simulink model "P702_NI_SoftECU"  (R2019a)
settings: Solver=ode1  StartTime=0.0  StopTime=Inf  FixedStep=0.001  RelTol=1e-3  EnableMultiTasking=on
PreLoadFcn:
  | run '.\VeriStand_BlockSet\NIVeriStandAddPaths.m'
undefined symbols (not defined in the file or in its folder): magnitude
libraries: simulink x83, simulink_extras x1
(part 1 of 76)
settings Model: Creator=HILTEST  LastModifiedBy=MSHI15
settings DataIOCC: LimitDataPoints=on  SaveFormat=Array  ReturnWorkspaceOutputs=off
settings OptimizationCC: BlockReduction=off  OptimizeBlockIOStorage=off  BufferReuse=off  GlobalBufferReuse=off  ExpressionFolding=off  LocalBlockOutputs=off  LifeSpan=inf  OptimizeDataStoreBuffers=off  BusAssignmentInplaceUpdate=off
settings DebuggingCC: InheritedTsInSrcMsg=none  RootOutportRequireBusObject=error  PregeneratedLibrarySubsystemCodeDiagnostic=none  StrictBusMsg=ErrorOnBusTreatedAsVector  SFUnexpectedBacktrackingDiag=warning  SFNoUnconditionalDefaultTransitionDiag=warning  SFExecutionAtInitializationDiag=none  ArithmeticOperatorsInVariantConditions=warning
settings HardwareCC: ProdBitPerPointer=32  ProdBitPerSizeT=32  ProdBitPerPtrDiffT=32  ProdLargestAtomicFloat=None  ProdWordSize=32  ProdHWDeviceType=Intel->x86/Pentium  TargetIntDivRoundTo=Zero  TargetEndianess=LittleEndian  TargetHWDeviceType=Generic->Custom
settings ModelReferenceCC: PropagateSignalLabelsOutOfModel=off
settings SFSimCC: SimUseLocalCustomCode=off
settings RTWCC: SystemTargetFile=NIVeriStand.tlc  TemplateMakefile=NIVeriStand_vc.tmf  Description=NI Phar Lap Real-Time & Windows Targets  RTWUseLocalCustomCode=off
settings CodeAppCC: StateflowObjectComments=on
settings STFCustomTargetCC: GeneratePreprocessorConditionals=Disable all  MatFileLogging=on  MATLABClassNameForMDSCustomization=Simulink.SoftwareTarget.TargetSpecificTriggerConfigurationBase  SystemTargetFile=NIVeriStand.tlc
settings ConfigComp: CovMetricSettings=dw  CovHtmlReporting=on  CovSaveCumulativeToWorkspaceVar=on  CovSaveSingleToWorkspaceVar=on  CovExternalEMLEnable=off

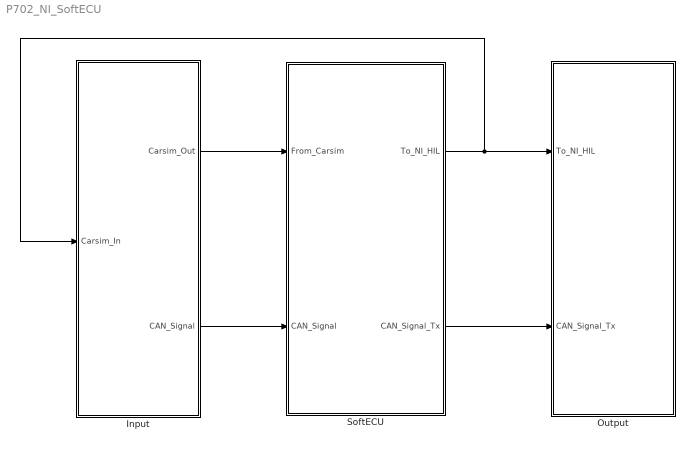
== system P702_NI_SoftECU ==
  Input : Subsystem
  Output : Subsystem
  SoftECU : Subsystem
  wires:
  SoftECU/1(To_NI_HIL) -> Input/1(Carsim_In), Output/1(To_NI_HIL)
  Input/1(Carsim_Out) -> SoftECU/1(From_Carsim)
  Input/2(CAN_Signal) -> SoftECU/2(CAN_Signal)
  SoftECU/2(CAN_Signal_Tx) -> Output/2(CAN_Signal_Tx)

== system P702_NI_SoftECU/Input ==
  Carsim_In : Inport
  ABS_ESC : Subsystem
  ABS_ESC_Disable : S-Function  Priority=1  FunctionName=NIVeriStandIO  Parameters=width dtype portnum stime stype btype  SFunctionDeploymentMode=off  EnableBusSupport=off  mask(NI VeriStand Inport){portnum=1, width=-1, stime=-1, dtype=auto, stype=auto, btype=1}
      mask prompts: portnum "Port number:"; width "Port dimensions (-1 for dynamically sized):"; stime "Sample time (-1 for inherited):"; dtype "Data type:"; stype "Signal type:"; btype "Block type:"
      mask help: Use this inport on any level of nested subsystems to allow NI VeriStand software to map signals to it.
      mask init:
      | NIVeriStandIO_init;
      settings: CopyFcn=NIVeriStand_MDL_functions('', 'IO_copy');  DeleteFcn=NIVeriStand_MDL_functions('', 'IO_delete');  MoveFcn=set_param(gcb, 'Mask', 'on');
      mask Callback portnum: NIVeriStand_MDL_functions('', 'IO_setportnum');
      mask TypeOptions dtype: auto | double | single | int8 | uint8 | int16 | uint16 | int32 | uint32 | boolean
      mask Callback dtype: NIVeriStand_MDL_functions('', 'IO_booleansignal');
      mask TypeOptions stype: auto | real | complex
      mask Display:
      | patch([-x x], [-y y], [.90980 .81960 .32156]);
      | plot([xrad -x x xrad], [yrad -y y yrad]);
      | fprintf('NI In%d', portnum);
  ADAS_Disable : S-Function  Priority=4  FunctionName=NIVeriStandIO  Parameters=width dtype portnum stime stype btype  SFunctionDeploymentMode=off  EnableBusSupport=off  mask(NI VeriStand Inport){portnum=4, width=-1, stime=-1, dtype=auto, stype=auto, btype=1}
      mask prompts: portnum "Port number:"; width "Port dimensions (-1 for dynamically sized):"; stime "Sample time (-1 for inherited):"; dtype "Data type:"; stype "Signal type:"; btype "Block type:"
      mask help: Use this inport on any level of nested subsystems to allow NI VeriStand software to map signals to it.
      mask init:
      | NIVeriStandIO_init;
      settings: CopyFcn=NIVeriStand_MDL_functions('', 'IO_copy');  DeleteFcn=NIVeriStand_MDL_functions('', 'IO_delete');  MoveFcn=set_param(gcb, 'Mask', 'on');
      mask Callback portnum: NIVeriStand_MDL_functions('', 'IO_setportnum');
      mask TypeOptions dtype: auto | double | single | int8 | uint8 | int16 | uint16 | int32 | uint32 | boolean
      mask Callback dtype: NIVeriStand_MDL_functions('', 'IO_booleansignal');
      mask TypeOptions stype: auto | real | complex
      mask Display:
      | patch([-x x], [-y y], [.90980 .81960 .32156]);
      | plot([xrad -x x xrad], [yrad -y y yrad]);
      | fprintf('NI In%d', portnum);
  BCM : Subsystem
  BCM_Disable : S-Function  Priority=3  FunctionName=NIVeriStandIO  Parameters=width dtype portnum stime stype btype  SFunctionDeploymentMode=off  EnableBusSupport=off  mask(NI VeriStand Inport){portnum=3, width=-1, stime=-1, dtype=auto, stype=auto, btype=1}
      mask prompts: portnum "Port number:"; width "Port dimensions (-1 for dynamically sized):"; stime "Sample time (-1 for inherited):"; dtype "Data type:"; stype "Signal type:"; btype "Block type:"
      mask help: Use this inport on any level of nested subsystems to allow NI VeriStand software to map signals to it.
      mask init:
      | NIVeriStandIO_init;
      settings: CopyFcn=NIVeriStand_MDL_functions('', 'IO_copy');  DeleteFcn=NIVeriStand_MDL_functions('', 'IO_delete');  MoveFcn=set_param(gcb, 'Mask', 'on');
      mask Callback portnum: NIVeriStand_MDL_functions('', 'IO_setportnum');
      mask TypeOptions dtype: auto | double | single | int8 | uint8 | int16 | uint16 | int32 | uint32 | boolean
      mask Callback dtype: NIVeriStand_MDL_functions('', 'IO_booleansignal');
      mask TypeOptions stype: auto | real | complex
      mask Display:
      | patch([-x x], [-y y], [.90980 .81960 .32156]);
      | plot([xrad -x x xrad], [yrad -y y yrad]);
      | fprintf('NI In%d', portnum);
  Bus_Ecu : BusCreator  Inputs=8
  Carsim : Subsystem
  DSMC : Subsystem
  DSMC_Disable : S-Function  Priority=6  FunctionName=NIVeriStandIO  Parameters=width dtype portnum stime stype btype  SFunctionDeploymentMode=off  EnableBusSupport=off  mask(NI VeriStand Inport){portnum=6, width=-1, stime=-1, dtype=auto, stype=auto, btype=1}
      mask prompts: portnum "Port number:"; width "Port dimensions (-1 for dynamically sized):"; stime "Sample time (-1 for inherited):"; dtype "Data type:"; stype "Signal type:"; btype "Block type:"
      mask help: Use this inport on any level of nested subsystems to allow NI VeriStand software to map signals to it.
      mask init:
      | NIVeriStandIO_init;
      settings: CopyFcn=NIVeriStand_MDL_functions('', 'IO_copy');  DeleteFcn=NIVeriStand_MDL_functions('', 'IO_delete');  MoveFcn=set_param(gcb, 'Mask', 'on');
      mask Callback portnum: NIVeriStand_MDL_functions('', 'IO_setportnum');
      mask TypeOptions dtype: auto | double | single | int8 | uint8 | int16 | uint16 | int32 | uint32 | boolean
      mask Callback dtype: NIVeriStand_MDL_functions('', 'IO_booleansignal');
      mask TypeOptions stype: auto | real | complex
      mask Display:
      | patch([-x x], [-y y], [.90980 .81960 .32156]);
      | plot([xrad -x x xrad], [yrad -y y yrad]);
      | fprintf('NI In%d', portnum);
  Display : Display
  ECM_DIESEL PCM PCM_HEV : Subsystem
  From_ADAS : Subsystem
  GWM-SCCM/PDB/RCM/GSM : Subsystem
  PCM_Disable : S-Function  Priority=5  FunctionName=NIVeriStandIO  Parameters=width dtype portnum stime stype btype  SFunctionDeploymentMode=off  EnableBusSupport=off  mask(NI VeriStand Inport){portnum=5, width=-1, stime=-1, dtype=auto, stype=auto, btype=1}
      mask prompts: portnum "Port number:"; width "Port dimensions (-1 for dynamically sized):"; stime "Sample time (-1 for inherited):"; dtype "Data type:"; stype "Signal type:"; btype "Block type:"
      mask help: Use this inport on any level of nested subsystems to allow NI VeriStand software to map signals to it.
      mask init:
      | NIVeriStandIO_init;
      settings: CopyFcn=NIVeriStand_MDL_functions('', 'IO_copy');  DeleteFcn=NIVeriStand_MDL_functions('', 'IO_delete');  MoveFcn=set_param(gcb, 'Mask', 'on');
      mask Callback portnum: NIVeriStand_MDL_functions('', 'IO_setportnum');
      mask TypeOptions dtype: auto | double | single | int8 | uint8 | int16 | uint16 | int32 | uint32 | boolean
      mask Callback dtype: NIVeriStand_MDL_functions('', 'IO_booleansignal');
      mask TypeOptions stype: auto | real | complex
      mask Display:
      | patch([-x x], [-y y], [.90980 .81960 .32156]);
      | plot([xrad -x x xrad], [yrad -y y yrad]);
      | fprintf('NI In%d', portnum);
  PSCM : Subsystem
  PSCM_Disable : S-Function  Priority=2  FunctionName=NIVeriStandIO  Parameters=width dtype portnum stime stype btype  SFunctionDeploymentMode=off  EnableBusSupport=off  mask(NI VeriStand Inport){portnum=2, width=-1, stime=-1, dtype=auto, stype=auto, btype=1}
      mask prompts: portnum "Port number:"; width "Port dimensions (-1 for dynamically sized):"; stime "Sample time (-1 for inherited):"; dtype "Data type:"; stype "Signal type:"; btype "Block type:"
      mask help: Use this inport on any level of nested subsystems to allow NI VeriStand software to map signals to it.
      mask init:
      | NIVeriStandIO_init;
      settings: CopyFcn=NIVeriStand_MDL_functions('', 'IO_copy');  DeleteFcn=NIVeriStand_MDL_functions('', 'IO_delete');  MoveFcn=set_param(gcb, 'Mask', 'on');
      mask Callback portnum: NIVeriStand_MDL_functions('', 'IO_setportnum');
      mask TypeOptions dtype: auto | double | single | int8 | uint8 | int16 | uint16 | int32 | uint32 | boolean
      mask Callback dtype: NIVeriStand_MDL_functions('', 'IO_booleansignal');
      mask TypeOptions stype: auto | real | complex
      mask Display:
      | patch([-x x], [-y y], [.90980 .81960 .32156]);
      | plot([xrad -x x xrad], [yrad -y y yrad]);
      | fprintf('NI In%d', portnum);
  RealPCM : Subsystem
  Carsim_Out : Outport
  CAN_Signal : Outport  Port=2
  wires:
  Carsim/1(Carsim_Out) -> Carsim_Out/1  "Carsim_Outl"
  PSCM/1(PSCM) -> Bus_Ecu/4  "PSCM"
  ECM_DIESEL PCM PCM_HEV/1(ECM_DIESEL PCM PCM_HEV) -> Bus_Ecu/5  "ECM_DIESEL PCM PCM_HEV"
  BCM/1(BCM) -> Bus_Ecu/6  "BCM"
  ABS_ESC_Disable/1 -> ABS_ESC/Enable
  PSCM_Disable/1 -> PSCM/Enable
  BCM_Disable/1 -> BCM/Enable
  From_ADAS/1(ADAS) -> Bus_Ecu/1  "ADAS"
  GWM-SCCM/PDB/RCM/GSM/1(GWM_FD1) -> Bus_Ecu/7  "GWM"
  PCM_Disable/1 -> ECM_DIESEL PCM PCM_HEV/Enable
  Bus_Ecu/1 -> CAN_Signal/1  "CAN_Signal"
  Carsim_In/1 -> Carsim/1(Carsim_In)
  ADAS_Disable/1 -> Display/1
  RealPCM/1(RealPCM) -> Bus_Ecu/2  "RealPCM"
  DSMC_Disable/1 -> DSMC/Enable
  DSMC/1(CMR_DSMC) -> Bus_Ecu/8  "DSMC"
  ABS_ESC/1(ABS_ESC) -> Bus_Ecu/3  "ABS_ESC"

== system P702_NI_SoftECU/Output ==
  To_NI_HIL : Inport
  CAN_Signal_Tx : Inport  Port=2
  ABS_ESC : Subsystem
  BCM : Subsystem
  Bus Selector : BusSelector  OutputSignals=ABS_ESC,PSCM,ECM_DIESEL PCM PCM_HEV,BCM,GWM,DSMC
  Bus Selector1 : BusSelector  OutputSignals=signal1,signal2
  BusCreator : BusCreator  Inputs=2
  DSMC : Subsystem
  ECM_DIESEL PCM PCM_HEV : Subsystem
  GWM : Subsystem
  PCAN_ADAS : Subsystem
  PSCM : Subsystem
  SoftECULogic_NIXNET_CAN_FD1 : Subsystem
  Subsystem : Subsystem
  Subsystem1 : Subsystem
  Subsystem2 : Subsystem
  wires:
  To_NI_HIL/1 -> BusCreator/1, PCAN_ADAS/1(In1), SoftECULogic_NIXNET_CAN_FD1/1(In1)
  Bus Selector/2 -> PSCM/1(PSCM_Tx)  "<PSCM>"
  Bus Selector/1 -> ABS_ESC/1(ABS_ESC_Tx)  "<ABS_ESC>"
  Bus Selector/3 -> ECM_DIESEL PCM PCM_HEV/1(ECM_DIESEL PCM PCM_HEV_Tx)  "<ECM_DIESEL PCM PCM_HEV>"
  Bus Selector/4 -> BCM/1(BCM_Tx)  "<BCM>"
  CAN_Signal_Tx/1 -> BusCreator/2, Bus Selector/1
  Bus Selector/5 -> GWM/1(GWM_Tx)  "<GWM>"
  Bus Selector/6 -> DSMC/1(DSMC)  "<DSMC>"
  BusCreator/1 -> Subsystem1/1(in_port), Bus Selector1/1

== system P702_NI_SoftECU/SoftECU ==
  From_Carsim : Inport
  CAN_Signal : Inport  Port=2
  ABS : Subsystem
  APIM : Subsystem
  BCM : Subsystem
  Bus Creator : BusCreator  Inputs=17
  Bus Selector : BusSelector  OutputSignals=ABS,PCM,ECM,TCM,PSCM,RCM,SCCM,MRR,BCM,SRR_R,SRR_L
  CCM : Subsystem
  DSMC : Subsystem
  ECM : Subsystem
  Ground{1..4} (4 alike) : Ground
  IPC : Subsystem
  IPMA : Subsystem
  MRR : Subsystem
  PCM : Subsystem
  PSCM : Subsystem
  RCM : Subsystem
  SCCM : Subsystem
  SRR_L : Subsystem
  SRR_R : Subsystem
  TCM : Subsystem
  To_NI_HIL : Outport
  CAN_Signal_Tx : Outport  Port=2
  wires:
  ABS/1(Out1) -> Bus Creator/1  "Soft_ABS"
  Bus Creator/1 -> To_NI_HIL/1  "To_NI_HIL"
  Bus Selector/1 -> ABS/1(In1)  "<ABS>"
  Bus Selector/2 -> PCM/1(In1)  "<PCM>"
  PCM/1(Out1) -> Bus Creator/2  "Soft_PCM"
  Bus Selector/3 -> ECM/1(In1)  "<ECM>"
  ECM/1(Out1) -> Bus Creator/3  "Soft_ECM"
  Bus Selector/4 -> PCM/3(In2), TCM/1(In1)  "<TCM>"
  TCM/1(Out1) -> Bus Creator/4  "Soft_TCM"
  Bus Selector/5 -> PSCM/1(In1)  "<PSCM>"
  PSCM/1(Out1) -> Bus Creator/5  "Soft_PSCM"
  Bus Selector/6 -> RCM/1(In1)  "<RCM>"
  RCM/1(Out1) -> Bus Creator/6  "Soft_RCM"
  Bus Selector/7 -> SCCM/1(In1)  "<SCCM>"
  SCCM/1(Out1) -> Bus Creator/7  "Soft_SCCM"
  MRR/1(Out1) -> Bus Creator/8  "Soft_MRR"
  IPC/1(Out1) -> Bus Creator/10  "Soft_IPC"
  APIM/1(Out1) -> Bus Creator/11  "Soft_APIM"
  IPMA/1(Out1) -> Bus Creator/12  "Soft_IPMA"
  CCM/1(Out1) -> Bus Creator/13  "Soft_CCM"
  From_Carsim/1 -> Bus Selector/1
  CAN_Signal/1 -> CAN_Signal_Tx/1, [CAN]
  Ground1/1 -> IPC/1(In1)
  Ground2/1 -> APIM/1(In1)
  Ground3/1 -> IPMA/1(In1)
  Ground4/1 -> CCM/1(In1)
  BCM/1(Out1) -> Bus Creator/9  "Soft_BCM"
  Bus Selector/9 -> BCM/1(In1)  "<BCM>"
  Bus Selector/8 -> Bus Creator/14, MRR/1(In1)  "<MRR>"
  [CAN] -> ECM/2(CAN), PCM/2(CAN), ABS/2(CAN)
  Bus Selector/10 -> SRR_R/1(In1)  "<SRR_R>"
  SRR_R/1(Out) -> Bus Creator/15  "SRR_R"
  Bus Selector/11 -> SRR_L/1(In1)  "<SRR_L>"
  SRR_L/1(Out) -> Bus Creator/16  "SRR_L"
  [CAN] -> DSMC/1(In1)
  DSMC/1(Out1) -> Bus Creator/17  "DSMC"

== system P702_NI_SoftECU/Input/ABS_ESC ==
  Enable : EnablePort
  ABS_AutoSar_NetworkMgt_0x596 : Subsystem
  ABS_BrkBst_Data_0x4B0 : Subsystem
  ABS_Rapid_Data_Response_1_0x6B0 : Subsystem
  ABS_Rapid_Data_Response_2_0x6B1 : Subsystem
  ActiveFronSteering_Req_0x88 : Subsystem
  BrakeSnData_3_0x77 : Subsystem
  BrakeSnData_4_0x7D : Subsystem
  BrakeSnData_5_0x76 : Subsystem
  BrakeSnData_6_0x414 : Subsystem
  BrakeSysFeatures_0x415 : Subsystem
  BrakeSysFeatures_2_0x416 : Subsystem
  BrakeSysFeatures_3_0x41E : Subsystem
  Bus_Msg : BusCreator  Inputs=22
  DesiredTorqBrk_0x213 : Subsystem
  DesiredTorqBrk_2_0x214 : Subsystem
  Global_PATS_SubTarget_0x49 : Subsystem
  SelectDriveModeData2_0x44E : Subsystem
  SelectDriveModeData_0x420 : Subsystem
  SteeringPinion_Data2_0x7F : Subsystem
  TesterPhysicalResABS_0x768 : Subsystem
  TrailerBrakeData_0x412 : Subsystem
  WheelData_0x216 : Subsystem
  WheelSpeed_0x217 : Subsystem
  ABS_ESC : Outport
  wires:
  BrakeSnData_5_0x76/1(BrakeSnData_5_0x76) -> Bus_Msg/2  "BrakeSnData_5_0x76"
  BrakeSysFeatures_2_0x416/1(BrakeSysFeatures_2_0x416) -> Bus_Msg/14  "BrakeSysFeatures_2_0x416"
  BrakeSysFeatures_0x415/1(BrakeSysFeatures_0x415) -> Bus_Msg/13  "BrakeSysFeatures_0x415"
  BrakeSnData_6_0x414/1(BrakeSnData_6_0x414) -> Bus_Msg/12  "BrakeSnData_6_0x414"
  TrailerBrakeData_0x412/1(TrailerBrakeData_0x412) -> Bus_Msg/11  "TrailerBrakeData_0x412"
  ABS_Rapid_Data_Response_2_0x6B1/1(ABS_Rapid_Data_Response_2_0x6B1) -> Bus_Msg/21  "ABS_Rapid_Data_Response_2_0x6B1"
  ABS_Rapid_Data_Response_1_0x6B0/1(ABS_Rapid_Data_Response_1_0x6B0) -> Bus_Msg/20  "ABS_Rapid_Data_Response_1_0x6B0"
  ABS_AutoSar_NetworkMgt_0x596/1(ABS_AutoSar_NetworkMgt_0x596) -> Bus_Msg/19  "ABS_AutoSar_NetworkMgt_0x596"
  ABS_BrkBst_Data_0x4B0/1(ABS_BrkBst_Data_0x4B0) -> Bus_Msg/18  "ABS_BrkBst_Data_0x4B0"
  SelectDriveModeData2_0x44E/1(SelectDriveModeData2_0x44E) -> Bus_Msg/17  "SelectDriveModeData2_0x44E"
  SelectDriveModeData_0x420/1(SelectDriveModeData_0x420) -> Bus_Msg/16  "SelectDriveModeData_0x420"
  BrakeSysFeatures_3_0x41E/1(BrakeSysFeatures_3_0x41E) -> Bus_Msg/15  "BrakeSysFeatures_3_0x41E"
  TesterPhysicalResABS_0x768/1(TesterPhysicalResABS_0x768) -> Bus_Msg/22  "TesterPhysicalResABS_0x768"
  WheelSpeed_0x217/1(WheelSpeed_0x217) -> Bus_Msg/10  "WheelSpeed_0x217"
  WheelData_0x216/1(WheelData_0x216) -> Bus_Msg/9  "WheelData_0x216"
  DesiredTorqBrk_2_0x214/1(DesiredTorqBrk_2_0x214) -> Bus_Msg/8  "DesiredTorqBrk_2_0x214"
  DesiredTorqBrk_0x213/1(DesiredTorqBrk_0x213) -> Bus_Msg/7  "DesiredTorqBrk_0x213"
  ActiveFronSteering_Req_0x88/1(ActiveFronSteering_Req_0x88) -> Bus_Msg/6  "ActiveFronSteering_Req_0x88"
  SteeringPinion_Data2_0x7F/1(SteeringPinion_Data2_0x7F) -> Bus_Msg/5  "SteeringPinion_Data2_0x7F"
  BrakeSnData_4_0x7D/1(BrakeSnData_4_0x7D) -> Bus_Msg/4  "BrakeSnData_4_0x7D"
  BrakeSnData_3_0x77/1(BrakeSnData_3_0x77) -> Bus_Msg/3  "BrakeSnData_3_0x77"
  Global_PATS_SubTarget_0x49/1(Global_PATS_SubTarget_0x49) -> Bus_Msg/1  "Global_PATS_SubTarget_0x49"
  Bus_Msg/1 -> ABS_ESC/1  "ABS_ESC"

== system P702_NI_SoftECU/Input/BCM ==
  Enable : EnablePort
  BCM_Lamp_Stat_0x3C3 : Subsystem
  Battery_Mgmt_24V_0x42E : Subsystem
  Battery_Mgmt_2_0x42C : Subsystem
  Battery_Mgmt_3_0x43C : Subsystem
  Battery_Mgmt_4_0x42B : Subsystem
  BodyInfo_3_0x3B3 : Subsystem
  Body_Info_10_0x3BA : Subsystem
  Body_Info_12_0x26E : Subsystem
  Body_Info_4_0x242 : Subsystem
  Body_Info_6_0x38D : Subsystem
  Body_Info_7_0x3B1 : Subsystem
  Body_Info_8_0x3B9 : Subsystem
  Body_Info_9_0x3A3 : Subsystem
  Bus_Msg : BusCreator  Inputs=30
  CMPS_FDM_Info_Status_0x3C7 : Subsystem
  CellPhonePassport_Stat_1_0x447 : Subsystem
  GGCC_Config_Mgmt_ID_1_0x40A : Subsystem
  GlobalClock_Data_0x84 : Subsystem
  Global_PATS_Control_Info2_0x42 : Subsystem
  Global_PATS_Control_Info_0x41 : Subsystem
  Locking_Systems_2_0x331 : Subsystem
  PaakRqData1_0x468 : Subsystem
  PaakRqData2_0x469 : Subsystem
  Personality_BCM2_Data_0x3EB : Subsystem
  Personality_BCM_Data_0x3E3 : Subsystem
  Power_Stat_0x456 : Subsystem
  RKE_Packet_0x3B6 : Subsystem
  TPM_Frame_0x3B7 : Subsystem
  Tire_Pressure_Data_0x3B5 : Subsystem
  Tire_Pressure_Data_DRW_0x3B8 : Subsystem
  Tire_Pressure_Stat_0x3B4 : Subsystem
  BCM : Outport
  wires:
  Bus_Msg/1 -> BCM/1  "BCM"
  Global_PATS_Control_Info_0x41/1(Global_PATS_Control_Info_0x41) -> Bus_Msg/1  "Global_PATS_Control_Info_0x41"
  Global_PATS_Control_Info2_0x42/1(Global_PATS_Control_Info2_0x42) -> Bus_Msg/2  "Global_PATS_Control_Info2_0x42"
  GlobalClock_Data_0x84/1(GlobalClock_Data_0x84) -> Bus_Msg/3  "GlobalClock_Data_0x84"
  Body_Info_4_0x242/1(Body_Info_4_0x242) -> Bus_Msg/4  "Body_Info_4_0x242"
  Body_Info_12_0x26E/1(Body_Info_12_0x26E) -> Bus_Msg/5  "Body_Info_12_0x26E"
  Locking_Systems_2_0x331/1(Locking_Systems_2_0x331) -> Bus_Msg/6  "Locking_Systems_2_0x331"
  Body_Info_6_0x38D/1(Body_Info_6_0x38D) -> Bus_Msg/7  "Body_Info_6_0x38D"
  Body_Info_9_0x3A3/1(Body_Info_9_0x3A3) -> Bus_Msg/8  "Body_Info_9_0x3A3"
  Body_Info_7_0x3B1/1(Body_Info_7_0x3B1) -> Bus_Msg/9  "Body_Info_7_0x3B1"
  BodyInfo_3_0x3B3/1(BodyInfo_3_0x3B3) -> Bus_Msg/10  "BodyInfo_3_0x3B3"
  Tire_Pressure_Stat_0x3B4/1(Tire_Pressure_Stat_0x3B4) -> Bus_Msg/11  "Tire_Pressure_Stat_0x3B4"
  Tire_Pressure_Data_0x3B5/1(Tire_Pressure_Data_0x3B5) -> Bus_Msg/12  "Tire_Pressure_Data_0x3B5"
  RKE_Packet_0x3B6/1(RKE_Packet_0x3B6) -> Bus_Msg/13  "RKE_Packet_0x3B6"
  TPM_Frame_0x3B7/1(TPM_Frame_0x3B7) -> Bus_Msg/14  "TPM_Frame_0x3B7"
  Tire_Pressure_Data_DRW_0x3B8/1(Tire_Pressure_Data_DRW_0x3B8) -> Bus_Msg/15  "Tire_Pressure_Data_DRW_0x3B8"
  Body_Info_8_0x3B9/1(Body_Info_8_0x3B9) -> Bus_Msg/16  "Body_Info_8_0x3B9"
  Body_Info_10_0x3BA/1(Body_Info_10_0x3BA) -> Bus_Msg/17  "Body_Info_10_0x3BA"
  BCM_Lamp_Stat_0x3C3/1(BCM_Lamp_Stat_0x3C3) -> Bus_Msg/18  "BCM_Lamp_Stat_0x3C3"
  CMPS_FDM_Info_Status_0x3C7/1(CMPS_FDM_Info_Status_0x3C7) -> Bus_Msg/19  "CMPS_FDM_Info_Status_0x3C7"
  Personality_BCM_Data_0x3E3/1(Personality_BCM_Data_0x3E3) -> Bus_Msg/20  "Personality_BCM_Data_0x3E3"
  Personality_BCM2_Data_0x3EB/1(Personality_BCM2_Data_0x3EB) -> Bus_Msg/21  "Personality_BCM2_Data_0x3EB"
  GGCC_Config_Mgmt_ID_1_0x40A/1(GGCC_Config_Mgmt_ID_1_0x40A) -> Bus_Msg/22  "GGCC_Config_Mgmt_ID_1_0x40A"
  Battery_Mgmt_4_0x42B/1(Battery_Mgmt_4_0x42B) -> Bus_Msg/23  "Battery_Mgmt_4_0x42B"
  Battery_Mgmt_2_0x42C/1(Battery_Mgmt_2_0x42C) -> Bus_Msg/24  "Battery_Mgmt_2_0x42C"
  Battery_Mgmt_24V_0x42E/1(Battery_Mgmt_24V_0x42E) -> Bus_Msg/25  "Battery_Mgmt_24V_0x42E"
  Battery_Mgmt_3_0x43C/1(Battery_Mgmt_3_0x43C) -> Bus_Msg/26  "Battery_Mgmt_3_0x43C"
  CellPhonePassport_Stat_1_0x447/1(CellPhonePassport_Stat_1_0x447) -> Bus_Msg/27  "CellPhonePassport_Stat_1_0x447"
  Power_Stat_0x456/1(Power_Stat_0x456) -> Bus_Msg/28  "Power_Stat_0x456"
  PaakRqData1_0x468/1(PaakRqData1_0x468) -> Bus_Msg/29  "PaakRqData1_0x468"
  PaakRqData2_0x469/1(PaakRqData2_0x469) -> Bus_Msg/30  "PaakRqData2_0x469"

== system P702_NI_SoftECU/Input/Carsim ==
  note: CarSim_SRR_L
  note: Bus Creators: Bus the signals coming from CarSim
  Carsim_In : Inport
  " CarSim_RCM" : Subsystem
  " CarSim_RCM2" : Subsystem  Commented=on
  BrakeActivation : Subsystem
  Bus Creator1 : BusCreator  Inputs=12
  Bus Conversion : Subsystem
  CarSimIn : S-Function  Priority=1  FunctionName=NIVeriStandIO  Parameters=width dtype portnum stime stype btype  SFunctionDeploymentMode=off  EnableBusSupport=off  mask(NI VeriStand Outport){portnum=1, width=-1, stime=-1, dtype=auto, stype=auto, btype=0}
      mask prompts: portnum "Port number:"; width "Port dimensions (-1 for dynamically sized):"; stime "Sample time (-1 for inherited):"; dtype "Data type:"; stype "Signal type:"; btype "Block type:"
      mask help: Use this outport on any level of nested subsystems to allow NI VeriStand software to map signals to it.
      mask init:
      | NIVeriStandIO_init;
      settings: CopyFcn=NIVeriStand_MDL_functions('', 'IO_copy');  DeleteFcn=NIVeriStand_MDL_functions('', 'IO_delete');  MoveFcn=set_param(gcb, 'Mask', 'on');
      mask Callback portnum: NIVeriStand_MDL_functions('', 'IO_setportnum');
      mask TypeOptions dtype: auto | double | single | int8 | uint8 | int16 | uint16 | int32 | uint32 | boolean
      mask Callback dtype: NIVeriStand_MDL_functions('', 'IO_booleansignal');
      mask TypeOptions stype: auto | real | complex
      mask Display:
      | patch([-x x], [-y y], [.90980 .81960 .32156]);
      | plot([xrad -x x xrad], [yrad -y y yrad]);
      | fprintf('NI Out%d', portnum);
  CarSim_ABS : Subsystem
  CarSim_ABS2 : Subsystem  Commented=on
  CarSim_BCM : Subsystem
  CarSim_BCM2 : Subsystem  Commented=on
  CarSim_ECM : Subsystem
  CarSim_ECM2 : Subsystem  Commented=on
  CarSim_GPSM : Subsystem
  CarSim_GPSM2 : Subsystem  Commented=on
  CarSim_MRR : Subsystem
  CarSim_MRR2 : Subsystem  Commented=on
  CarSim_PCM : Subsystem
  CarSim_PCM2 : Subsystem  Commented=on
  CarSim_PSCM : Subsystem
  CarSim_PSCM2 : Subsystem  Commented=on
  CarSim_SCCM : Subsystem
  CarSim_SCCM2 : Subsystem  Commented=on
  CarSim_SRR_L : Subsystem
  CarSim_SRR_R : Subsystem
  CarSim_TCM : Subsystem
  CarSim_TCM2 : Subsystem  Commented=on
  SystemSetting : Subsystem
  Carsim_Out : Outport
  wires:
  CarSim_BCM/1(Out1) -> Bus Creator1/9
  CarSim_SCCM/1(Out1) -> Bus Creator1/7
  CarSim_PSCM/1(Out1) -> Bus Creator1/5
  CarSim_ECM/1(Out1) -> Bus Creator1/3
  CarSim_PCM/1(Out1) -> Bus Creator1/2
  CarSim_GPSM/1(Out1) -> Bus Creator1/8
  " CarSim_RCM"/1(Out1) -> Bus Creator1/6
  CarSim_TCM/1(Out1) -> Bus Creator1/4
  CarSim_MRR/1(Out1) -> Bus Creator1/10
  CarSim_ABS/1(Out2) -> Bus Creator1/1
  Carsim_In/1 -> BrakeActivation/1(In1)
  BrakeActivation/1(Out1) -> CarSimIn/1
  Bus Conversion/1(to Model) -> Carsim_Out/1
  Bus Creator1/1 -> Bus Conversion/1(From CarSim S-Function)
  CarSim_SRR_L/1(Out1) -> Bus Creator1/12
  CarSim_SRR_R/1(Out1) -> Bus Creator1/11

== system P702_NI_SoftECU/Input/DSMC ==
  Enable : EnablePort
  Bus_Msg : BusCreator  Inputs=3
  CMR_DSMC_AutoSar_NetwrkMgt : Subsystem
  DrvStatMonData : Subsystem
  TesterPhysicalResCMR_DSMC : Subsystem
  CMR_DSMC : Outport
  wires:
  Bus_Msg/1 -> CMR_DSMC/1  "DSMC"
  CMR_DSMC_AutoSar_NetwrkMgt/1(CMR_DSMC_AutoSar_NetwrkMgt_5DF) -> Bus_Msg/1  "CMR_DSMC_AutoSar_NetwrkMgt"
  DrvStatMonData/1(DrvStatMonData_450) -> Bus_Msg/2  "DrvStatMonData"
  TesterPhysicalResCMR_DSMC/1(TesterPhysicalResCMR_DSMC_7C9) -> Bus_Msg/3  "TesterPhysicalResCMR_DSMC"

== system P702_NI_SoftECU/Input/ECM_DIESEL PCM PCM_HEV ==
  Enable : EnablePort
  Bus_Msg : BusCreator  Inputs=26
  EngBrakeData_0x165 : Subsystem
  EngVehicleSpThrottle2_0x202 : Subsystem
  EngVehicleSpThrottle_0x204 : Subsystem
  EngineClimateData_0x178 : Subsystem
  EngineData_6_0x156 : Subsystem
  EngineData_7_0x179 : Subsystem
  Engine_Clutch_Data_0x42F : Subsystem
  Gear_Shift_by_Wire_3 : Subsystem
  Global_PATS_TargetInfo_0x47 : Subsystem
  HEV_Powertrain_Data2 : Subsystem
  PCM_AutoSar_NetworkMgmt_0x595 : Subsystem
  PCM_Rapid_Data_Response_1_0x6A0 : Subsystem
  PowertrainData_10 : Subsystem
  PowertrainData_1_0x421 : Subsystem
  PowertrainData_2_0x42D : Subsystem
  PowertrainData_3_0x43E : Subsystem
  PowertrainData_6_0x205 : Subsystem
  PowertrainData_7_0x41F : Subsystem
  PowertrainData_9_0x44C : Subsystem
  Powertrain_Data_4_0x424 : Subsystem
  Powertrain_Data_5_0x43F : Subsystem
  Stop_Start_0x166 : Subsystem
  TesterPhysicalResPCM_0x7E8 : Subsystem
  TorqueDataEngFlags_0x200 : Subsystem
  TransGearData : Subsystem
  VehicleOperatingModes_0x167 : Subsystem
  ECM_DIESEL PCM PCM_HEV : Outport
  wires:
  Bus_Msg/1 -> ECM_DIESEL PCM PCM_HEV/1  "ECM_DIESEL PCM PCM_HEV"
  Global_PATS_TargetInfo_0x47/1(Global_PATS_TargetInfo_0x47) -> Bus_Msg/1  "Global_PATS_TargetInfo_0x47"
  EngineData_6_0x156/1(EngineData_6_0x156) -> Bus_Msg/2  "EngineData_6_0x156"
  EngBrakeData_0x165/1(EngBrakeData_0x165) -> Bus_Msg/3  "EngBrakeData_0x165"
  Stop_Start_0x166/1(Stop_Start_0x166) -> Bus_Msg/4  "Stop_Start_0x166"
  VehicleOperatingModes_0x167/1(VehicleOperatingModes_0x167) -> Bus_Msg/5  "VehicleOperatingModes_0x167"
  EngineClimateData_0x178/1(EngineClimateData_0x178) -> Bus_Msg/6  "EngineClimateData_0x178"
  EngineData_7_0x179/1(EngineData_7_0x179) -> Bus_Msg/7  "EngineData_7_0x179"
  TorqueDataEngFlags_0x200/1(TorqueDataEngFlags_0x200) -> Bus_Msg/8  "TorqueDataEngFlags_0x200"
  EngVehicleSpThrottle2_0x202/1(EngVehicleSpThrottle2_0x202) -> Bus_Msg/9  "EngVehicleSpThrottle2_0x202"
  EngVehicleSpThrottle_0x204/1(EngVehicleSpThrottle_0x204) -> Bus_Msg/10  "EngVehicleSpThrottle_0x204"
  PowertrainData_6_0x205/1(PowertrainData_6_0x205) -> Bus_Msg/11  "PowertrainData_6_0x205"
  PowertrainData_7_0x41F/1(PowertrainData_7_0x41F) -> Bus_Msg/12  "PowertrainData_7_0x41F"
  PowertrainData_1_0x421/1(PowertrainData_1_0x421) -> Bus_Msg/13  "PowertrainData_1_0x421"
  Powertrain_Data_4_0x424/1(Powertrain_Data_4_0x424) -> Bus_Msg/14  "Powertrain_Data_4_0x424"
  PowertrainData_2_0x42D/1(PowertrainData_2_0x42D) -> Bus_Msg/15  "PowertrainData_2_0x42D"
  Engine_Clutch_Data_0x42F/1(Engine_Clutch_Data_0x42F) -> Bus_Msg/16  "Engine_Clutch_Data_0x42F"
  PowertrainData_3_0x43E/1(PowertrainData_3_0x43E) -> Bus_Msg/17  "PowertrainData_3_0x43E"
  Powertrain_Data_5_0x43F/1(Powertrain_Data_5_0x43F) -> Bus_Msg/18  "Powertrain_Data_5_0x43F"
  PowertrainData_9_0x44C/1(PowertrainData_9_0x44C) -> Bus_Msg/19  "PowertrainData_9_0x44C"
  PCM_AutoSar_NetworkMgmt_0x595/1(PCM_AutoSar_NetworkMgmt_0x595) -> Bus_Msg/20  "PCM_AutoSar_NetworkMgmt_0x595"
  PCM_Rapid_Data_Response_1_0x6A0/1(PCM_Rapid_Data_Response_1_0x6A0) -> Bus_Msg/21  "PCM_Rapid_Data_Response_1_0x6A0"
  TesterPhysicalResPCM_0x7E8/1(TesterPhysicalResPCM_0x7E8) -> Bus_Msg/22  "TesterPhysicalResPCM_0x7E8"
  Gear_Shift_by_Wire_3/1(Gear_Shift_by_Wire_3_5C) -> Bus_Msg/23  "Gear_Shift_by_Wire_3"
  PowertrainData_10/1(PowertrainData_10_176) -> Bus_Msg/24  "PowertrainData_10"
  TransGearData/1(TransGearData_230) -> Bus_Msg/25  "TransGearData"
  HEV_Powertrain_Data2/1(HEV_Powertrain_Data2_25B) -> Bus_Msg/26  "HEV_Powertrain_Data2"

== system P702_NI_SoftECU/Input/From_ADAS ==
  ACCBrkDecel_B_Rq : S-Function  Priority=1  FunctionName=NIVeriStandIO  Parameters=width dtype portnum stime stype btype  SFunctionDeploymentMode=off  EnableBusSupport=off  mask(NI VeriStand Inport){portnum=1, width=1, stime=-1, dtype=auto, stype=auto, btype=1}
      mask prompts: portnum "Port number:"; width "Port dimensions (-1 for dynamically sized):"; stime "Sample time (-1 for inherited):"; dtype "Data type:"; stype "Signal type:"; btype "Block type:"
      mask help: Use this inport on any level of nested subsystems to allow NI VeriStand software to map signals to it.
      mask init:
      | NIVeriStandIO_init;
      settings: CopyFcn=NIVeriStand_MDL_functions('', 'IO_copy');  DeleteFcn=NIVeriStand_MDL_functions('', 'IO_delete');  MoveFcn=set_param(gcb, 'Mask', 'on');
      mask Callback portnum: NIVeriStand_MDL_functions('', 'IO_setportnum');
      mask TypeOptions dtype: auto | double | single | int8 | uint8 | int16 | uint16 | int32 | uint32 | boolean
      mask Callback dtype: NIVeriStand_MDL_functions('', 'IO_booleansignal');
      mask TypeOptions stype: auto | real | complex
      mask Display:
      | patch([-x x], [-y y], [.90980 .81960 .32156]);
      | plot([xrad -x x xrad], [yrad -y y yrad]);
      | fprintf('NI In%d', portnum);
  AccBrkPrchg_B_Rq : S-Function  Priority=2  FunctionName=NIVeriStandIO  Parameters=width dtype portnum stime stype btype  SFunctionDeploymentMode=off  EnableBusSupport=off  mask(NI VeriStand Inport){portnum=2, width=1, stime=-1, dtype=auto, stype=auto, btype=1}
      mask prompts: portnum "Port number:"; width "Port dimensions (-1 for dynamically sized):"; stime "Sample time (-1 for inherited):"; dtype "Data type:"; stype "Signal type:"; btype "Block type:"
      mask help: Use this inport on any level of nested subsystems to allow NI VeriStand software to map signals to it.
      mask init:
      | NIVeriStandIO_init;
      settings: CopyFcn=NIVeriStand_MDL_functions('', 'IO_copy');  DeleteFcn=NIVeriStand_MDL_functions('', 'IO_delete');  MoveFcn=set_param(gcb, 'Mask', 'on');
      mask Callback portnum: NIVeriStand_MDL_functions('', 'IO_setportnum');
      mask TypeOptions dtype: auto | double | single | int8 | uint8 | int16 | uint16 | int32 | uint32 | boolean
      mask Callback dtype: NIVeriStand_MDL_functions('', 'IO_booleansignal');
      mask TypeOptions stype: auto | real | complex
      mask Display:
      | patch([-x x], [-y y], [.90980 .81960 .32156]);
      | plot([xrad -x x xrad], [yrad -y y yrad]);
      | fprintf('NI In%d', portnum);
  AccBrkTot_A_Rq : S-Function  Priority=4  FunctionName=NIVeriStandIO  Parameters=width dtype portnum stime stype btype  SFunctionDeploymentMode=off  EnableBusSupport=off  mask(NI VeriStand Inport){portnum=4, width=1, stime=-1, dtype=auto, stype=auto, btype=1}
      mask prompts: portnum "Port number:"; width "Port dimensions (-1 for dynamically sized):"; stime "Sample time (-1 for inherited):"; dtype "Data type:"; stype "Signal type:"; btype "Block type:"
      mask help: Use this inport on any level of nested subsystems to allow NI VeriStand software to map signals to it.
      mask init:
      | NIVeriStandIO_init;
      settings: CopyFcn=NIVeriStand_MDL_functions('', 'IO_copy');  DeleteFcn=NIVeriStand_MDL_functions('', 'IO_delete');  MoveFcn=set_param(gcb, 'Mask', 'on');
      mask Callback portnum: NIVeriStand_MDL_functions('', 'IO_setportnum');
      mask TypeOptions dtype: auto | double | single | int8 | uint8 | int16 | uint16 | int32 | uint32 | boolean
      mask Callback dtype: NIVeriStand_MDL_functions('', 'IO_booleansignal');
      mask TypeOptions stype: auto | real | complex
      mask Display:
      | patch([-x x], [-y y], [.90980 .81960 .32156]);
      | plot([xrad -x x xrad], [yrad -y y yrad]);
      | fprintf('NI In%d', portnum);
  AccCancl_B_Rq : S-Function  Priority=10  FunctionName=NIVeriStandIO  Parameters=width dtype portnum stime stype btype  SFunctionDeploymentMode=off  EnableBusSupport=off  mask(NI VeriStand Inport){portnum=10, width=1, stime=-1, dtype=auto, stype=auto, btype=1}
      mask prompts: portnum "Port number:"; width "Port dimensions (-1 for dynamically sized):"; stime "Sample time (-1 for inherited):"; dtype "Data type:"; stype "Signal type:"; btype "Block type:"
      mask help: Use this inport on any level of nested subsystems to allow NI VeriStand software to map signals to it.
      mask init:
      | NIVeriStandIO_init;
      settings: CopyFcn=NIVeriStand_MDL_functions('', 'IO_copy');  DeleteFcn=NIVeriStand_MDL_functions('', 'IO_delete');  MoveFcn=set_param(gcb, 'Mask', 'on');
      mask Callback portnum: NIVeriStand_MDL_functions('', 'IO_setportnum');
      mask TypeOptions dtype: auto | double | single | int8 | uint8 | int16 | uint16 | int32 | uint32 | boolean
      mask Callback dtype: NIVeriStand_MDL_functions('', 'IO_booleansignal');
      mask TypeOptions stype: auto | real | complex
      mask Display:
      | patch([-x x], [-y y], [.90980 .81960 .32156]);
      | plot([xrad -x x xrad], [yrad -y y yrad]);
      | fprintf('NI In%d', portnum);
  AccPrpl_A_Rq : S-Function  Priority=11  FunctionName=NIVeriStandIO  Parameters=width dtype portnum stime stype btype  SFunctionDeploymentMode=off  EnableBusSupport=off  mask(NI VeriStand Inport){portnum=11, width=1, stime=-1, dtype=auto, stype=auto, btype=1}
      mask prompts: portnum "Port number:"; width "Port dimensions (-1 for dynamically sized):"; stime "Sample time (-1 for inherited):"; dtype "Data type:"; stype "Signal type:"; btype "Block type:"
      mask help: Use this inport on any level of nested subsystems to allow NI VeriStand software to map signals to it.
      mask init:
      | NIVeriStandIO_init;
      settings: CopyFcn=NIVeriStand_MDL_functions('', 'IO_copy');  DeleteFcn=NIVeriStand_MDL_functions('', 'IO_delete');  MoveFcn=set_param(gcb, 'Mask', 'on');
      mask Callback portnum: NIVeriStand_MDL_functions('', 'IO_setportnum');
      mask TypeOptions dtype: auto | double | single | int8 | uint8 | int16 | uint16 | int32 | uint32 | boolean
      mask Callback dtype: NIVeriStand_MDL_functions('', 'IO_booleansignal');
      mask TypeOptions stype: auto | real | complex
      mask Display:
      | patch([-x x], [-y y], [.90980 .81960 .32156]);
      | plot([xrad -x x xrad], [yrad -y y yrad]);
      | fprintf('NI In%d', portnum);
  AccPrpl_A_Rq1 : S-Function  Priority=12  FunctionName=NIVeriStandIO  Parameters=width dtype portnum stime stype btype  SFunctionDeploymentMode=off  EnableBusSupport=off  mask(NI VeriStand Inport){portnum=12, width=1, stime=-1, dtype=auto, stype=auto, btype=1}
      mask prompts: portnum "Port number:"; width "Port dimensions (-1 for dynamically sized):"; stime "Sample time (-1 for inherited):"; dtype "Data type:"; stype "Signal type:"; btype "Block type:"
      mask help: Use this inport on any level of nested subsystems to allow NI VeriStand software to map signals to it.
      mask init:
      | NIVeriStandIO_init;
      settings: CopyFcn=NIVeriStand_MDL_functions('', 'IO_copy');  DeleteFcn=NIVeriStand_MDL_functions('', 'IO_delete');  MoveFcn=set_param(gcb, 'Mask', 'on');
      mask Callback portnum: NIVeriStand_MDL_functions('', 'IO_setportnum');
      mask TypeOptions dtype: auto | double | single | int8 | uint8 | int16 | uint16 | int32 | uint32 | boolean
      mask Callback dtype: NIVeriStand_MDL_functions('', 'IO_booleansignal');
      mask TypeOptions stype: auto | real | complex
      mask Display:
      | patch([-x x], [-y y], [.90980 .81960 .32156]);
      | plot([xrad -x x xrad], [yrad -y y yrad]);
      | fprintf('NI In%d', portnum);
  AccStopStat_B_Rq : S-Function  Priority=3  FunctionName=NIVeriStandIO  Parameters=width dtype portnum stime stype btype  SFunctionDeploymentMode=off  EnableBusSupport=off  mask(NI VeriStand Inport){portnum=3, width=1, stime=-1, dtype=auto, stype=auto, btype=1}
      mask prompts: portnum "Port number:"; width "Port dimensions (-1 for dynamically sized):"; stime "Sample time (-1 for inherited):"; dtype "Data type:"; stype "Signal type:"; btype "Block type:"
      mask help: Use this inport on any level of nested subsystems to allow NI VeriStand software to map signals to it.
      mask init:
      | NIVeriStandIO_init;
      settings: CopyFcn=NIVeriStand_MDL_functions('', 'IO_copy');  DeleteFcn=NIVeriStand_MDL_functions('', 'IO_delete');  MoveFcn=set_param(gcb, 'Mask', 'on');
      mask Callback portnum: NIVeriStand_MDL_functions('', 'IO_setportnum');
      mask TypeOptions dtype: auto | double | single | int8 | uint8 | int16 | uint16 | int32 | uint32 | boolean
      mask Callback dtype: NIVeriStand_MDL_functions('', 'IO_booleansignal');
      mask TypeOptions stype: auto | real | complex
      mask Display:
      | patch([-x x], [-y y], [.90980 .81960 .32156]);
      | plot([xrad -x x xrad], [yrad -y y yrad]);
      | fprintf('NI In%d', portnum);
  Bus Creator : BusCreator  Inputs=8
  Bus Creator1 : BusCreator  Inputs=4
  Bus Creator2 : BusCreator  Inputs=2
  CmbbBaSens_D_Rq : S-Function  Priority=8  FunctionName=NIVeriStandIO  Parameters=width dtype portnum stime stype btype  SFunctionDeploymentMode=off  EnableBusSupport=off  mask(NI VeriStand Inport){portnum=8, width=1, stime=-1, dtype=auto, stype=auto, btype=1}
      mask prompts: portnum "Port number:"; width "Port dimensions (-1 for dynamically sized):"; stime "Sample time (-1 for inherited):"; dtype "Data type:"; stype "Signal type:"; btype "Block type:"
      mask help: Use this inport on any level of nested subsystems to allow NI VeriStand software to map signals to it.
      mask init:
      | NIVeriStandIO_init;
      settings: CopyFcn=NIVeriStand_MDL_functions('', 'IO_copy');  DeleteFcn=NIVeriStand_MDL_functions('', 'IO_delete');  MoveFcn=set_param(gcb, 'Mask', 'on');
      mask Callback portnum: NIVeriStand_MDL_functions('', 'IO_setportnum');
      mask TypeOptions dtype: auto | double | single | int8 | uint8 | int16 | uint16 | int32 | uint32 | boolean
      mask Callback dtype: NIVeriStand_MDL_functions('', 'IO_booleansignal');
      mask TypeOptions stype: auto | real | complex
      mask Display:
      | patch([-x x], [-y y], [.90980 .81960 .32156]);
      | plot([xrad -x x xrad], [yrad -y y yrad]);
      | fprintf('NI In%d', portnum);
  CmbbBrkDecel_A_Rq : S-Function  Priority=5  FunctionName=NIVeriStandIO  Parameters=width dtype portnum stime stype btype  SFunctionDeploymentMode=off  EnableBusSupport=off  mask(NI VeriStand Inport){portnum=5, width=1, stime=-1, dtype=auto, stype=auto, btype=1}
      mask prompts: portnum "Port number:"; width "Port dimensions (-1 for dynamically sized):"; stime "Sample time (-1 for inherited):"; dtype "Data type:"; stype "Signal type:"; btype "Block type:"
      mask help: Use this inport on any level of nested subsystems to allow NI VeriStand software to map signals to it.
      mask init:
      | NIVeriStandIO_init;
      settings: CopyFcn=NIVeriStand_MDL_functions('', 'IO_copy');  DeleteFcn=NIVeriStand_MDL_functions('', 'IO_delete');  MoveFcn=set_param(gcb, 'Mask', 'on');
      mask Callback portnum: NIVeriStand_MDL_functions('', 'IO_setportnum');
      mask TypeOptions dtype: auto | double | single | int8 | uint8 | int16 | uint16 | int32 | uint32 | boolean
      mask Callback dtype: NIVeriStand_MDL_functions('', 'IO_booleansignal');
      mask TypeOptions stype: auto | real | complex
      mask Display:
      | patch([-x x], [-y y], [.90980 .81960 .32156]);
      | plot([xrad -x x xrad], [yrad -y y yrad]);
      | fprintf('NI In%d', portnum);
  CmbbBrkDecel_B_Rq : S-Function  Priority=7  FunctionName=NIVeriStandIO  Parameters=width dtype portnum stime stype btype  SFunctionDeploymentMode=off  EnableBusSupport=off  mask(NI VeriStand Inport){portnum=7, width=1, stime=-1, dtype=auto, stype=auto, btype=1}
      mask prompts: portnum "Port number:"; width "Port dimensions (-1 for dynamically sized):"; stime "Sample time (-1 for inherited):"; dtype "Data type:"; stype "Signal type:"; btype "Block type:"
      mask help: Use this inport on any level of nested subsystems to allow NI VeriStand software to map signals to it.
      mask init:
      | NIVeriStandIO_init;
      settings: CopyFcn=NIVeriStand_MDL_functions('', 'IO_copy');  DeleteFcn=NIVeriStand_MDL_functions('', 'IO_delete');  MoveFcn=set_param(gcb, 'Mask', 'on');
      mask Callback portnum: NIVeriStand_MDL_functions('', 'IO_setportnum');
      mask TypeOptions dtype: auto | double | single | int8 | uint8 | int16 | uint16 | int32 | uint32 | boolean
      mask Callback dtype: NIVeriStand_MDL_functions('', 'IO_booleansignal');
      mask TypeOptions stype: auto | real | complex
      mask Display:
      | patch([-x x], [-y y], [.90980 .81960 .32156]);
      | plot([xrad -x x xrad], [yrad -y y yrad]);
      | fprintf('NI In%d', portnum);
  CmbbBrkPrchg_D_Rq : S-Function  Priority=6  FunctionName=NIVeriStandIO  Parameters=width dtype portnum stime stype btype  SFunctionDeploymentMode=off  EnableBusSupport=off  mask(NI VeriStand Inport){portnum=6, width=1, stime=-1, dtype=auto, stype=auto, btype=1}
      mask prompts: portnum "Port number:"; width "Port dimensions (-1 for dynamically sized):"; stime "Sample time (-1 for inherited):"; dtype "Data type:"; stype "Signal type:"; btype "Block type:"
      mask help: Use this inport on any level of nested subsystems to allow NI VeriStand software to map signals to it.
      mask init:
      | NIVeriStandIO_init;
      settings: CopyFcn=NIVeriStand_MDL_functions('', 'IO_copy');  DeleteFcn=NIVeriStand_MDL_functions('', 'IO_delete');  MoveFcn=set_param(gcb, 'Mask', 'on');
      mask Callback portnum: NIVeriStand_MDL_functions('', 'IO_setportnum');
      mask TypeOptions dtype: auto | double | single | int8 | uint8 | int16 | uint16 | int32 | uint32 | boolean
      mask Callback dtype: NIVeriStand_MDL_functions('', 'IO_booleansignal');
      mask TypeOptions stype: auto | real | complex
      mask Display:
      | patch([-x x], [-y y], [.90980 .81960 .32156]);
      | plot([xrad -x x xrad], [yrad -y y yrad]);
      | fprintf('NI In%d', portnum);
  CmbbEngTqMn_B_Rq : S-Function  Priority=9  FunctionName=NIVeriStandIO  Parameters=width dtype portnum stime stype btype  SFunctionDeploymentMode=off  EnableBusSupport=off  mask(NI VeriStand Inport){portnum=9, width=1, stime=-1, dtype=auto, stype=auto, btype=1}
      mask prompts: portnum "Port number:"; width "Port dimensions (-1 for dynamically sized):"; stime "Sample time (-1 for inherited):"; dtype "Data type:"; stype "Signal type:"; btype "Block type:"
      mask help: Use this inport on any level of nested subsystems to allow NI VeriStand software to map signals to it.
      mask init:
      | NIVeriStandIO_init;
      settings: CopyFcn=NIVeriStand_MDL_functions('', 'IO_copy');  DeleteFcn=NIVeriStand_MDL_functions('', 'IO_delete');  MoveFcn=set_param(gcb, 'Mask', 'on');
      mask Callback portnum: NIVeriStand_MDL_functions('', 'IO_setportnum');
      mask TypeOptions dtype: auto | double | single | int8 | uint8 | int16 | uint16 | int32 | uint32 | boolean
      mask Callback dtype: NIVeriStand_MDL_functions('', 'IO_booleansignal');
      mask TypeOptions stype: auto | real | complex
      mask Display:
      | patch([-x x], [-y y], [.90980 .81960 .32156]);
      | plot([xrad -x x xrad], [yrad -y y yrad]);
      | fprintf('NI In%d', portnum);
  ADAS : Outport
  wires:
  ACCBrkDecel_B_Rq/1 -> Bus Creator/2  "AccBrkDecel_B_Rq"
  AccBrkTot_A_Rq/1 -> Bus Creator/4  "AccBrkTot_A_Rq"
  AccStopStat_B_Rq/1 -> Bus Creator/3  "AccStopStat_B_Rq"
  AccBrkPrchg_B_Rq/1 -> Bus Creator/1  "AccBrkPrchg_B_Rq"
  CmbbBrkDecel_A_Rq/1 -> Bus Creator1/2  "CmbbBrkDecel_A_Rq"
  CmbbBrkDecel_B_Rq/1 -> Bus Creator1/4  "CmbbBrkDecel_B_Rq"
  CmbbBaSens_D_Rq/1 -> Bus Creator1/3  "CmbbBaSens_D_Rq"
  CmbbBrkPrchg_D_Rq/1 -> Bus Creator1/1  "CmbbBrkPrchg_D_Rq"
  Bus Creator/1 -> Bus Creator2/1  "ACCDATA"
  Bus Creator1/1 -> Bus Creator2/2  "ACCDATA_2"
  Bus Creator2/1 -> ADAS/1  "ADAS"
  CmbbEngTqMn_B_Rq/1 -> Bus Creator/5  "CmbbEngTqMn_B_Rq"
  AccPrpl_A_Rq/1 -> Bus Creator/7  "AccPrpl_A_Rq"
  AccCancl_B_Rq/1 -> Bus Creator/6  "AccCancl_B_Rq"
  AccPrpl_A_Rq1/1 -> Bus Creator/8  "AccPrpl_A_Rq1"
